simulink model "test"  (R2017b)
settings: Solver=VariableStepAuto  StartTime=0.0  StopTime=15  RelTol=1e-3
libraries: simulink x1
settings Model: Creator=Administrator  LastModifiedBy=Administrator

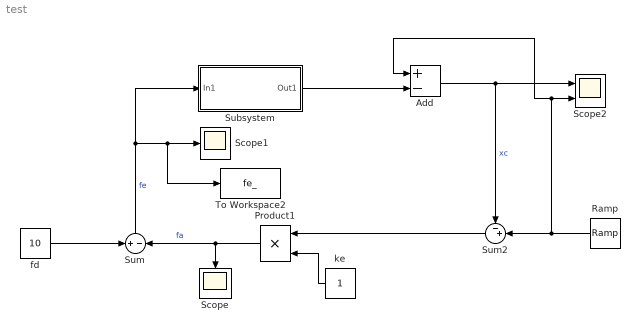
== system test ==
  Add : Sum  Inputs=+-
  Product1 : Product
  Ramp : simulink/Sources/Ramp  slope=0.1  start=0  X0=0
  Scope : Scope
  Scope1 : Scope
  Scope2 : Scope  NumInputPorts=2
  Subsystem : Subsystem
  Sum : Sum  Inputs=+|-
  Sum2 : Sum  Inputs=-+|
  To Workspace2 : ToWorkspace  VariableName=fe_  SampleTime=0.01
      settings: Save2DSignal=2-D array (concatenate along first dimension)
  fd : Constant  Value=10
  ke : Constant
  wires:
  Subsystem/1(Out1) -> Add/2
  Ramp/1 -> Add/1, Scope2/2, Sum2/2
  ke/1 -> Product1/2
  Product1/1 -> Sum/2, Scope/1  "fa"
  fd/1 -> Sum/1
  Sum/1 -> Subsystem/1(In1), To Workspace2/1, Scope1/1  "fe"
  Sum2/1 -> Product1/1
  Add/1 -> Scope2/1, Sum2/1  "xc"

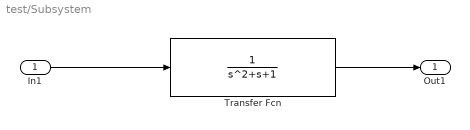
== system test/Subsystem ==
  In1 : Inport
  Transfer Fcn : TransferFcn  Denominator=[1 1 1]
  Out1 : Outport
  wires:
  In1/1 -> Transfer Fcn/1
  Transfer Fcn/1 -> Out1/1
